simulink model "chap7_2sim_Sfunction"  (R2014b)
settings: Solver=ode45  StartTime=0.0  StopTime=10  RelTol=1e-3
libraries: fod x2
settings Model: ExtModeTrigMode=oneshot  ExtModeArmWhenConnect=off  Creator=Administrator  LastModifiedBy=Administrator
settings DataIOCC: LimitDataPoints=off  SignalLoggingSaveFormat=ModelDataLogs  SignalLoggingName=sigsOut
settings OptimizationCC: BooleanDataType=off
settings DebuggingCC: SaveWithParameterizedLinksMsg=none  UnderspecifiedInitializationDetection=Classic  MergeDetectMultiDrivingBlocksExec=none  SignalResolutionControl=TryResolveAllWithWarning  SolverPrmCheckMsg=none  MultiTaskDSMMsg=warning  MultiTaskCondExecSysMsg=none
settings HardwareCC: TargetUnknown=on
settings RTWCC: IncludeERTFirstTime=on
settings GRTTargetCC: CombineOutputUpdateFcns=off  GRTInterface=on

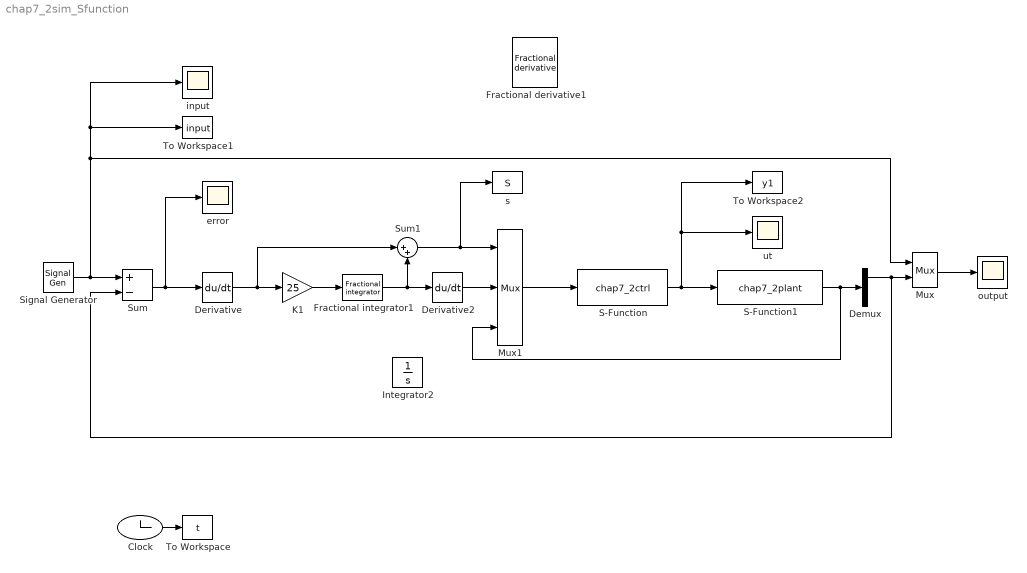
== system chap7_2sim_Sfunction ==
  Clock : Clock
  Demux : Demux  Outputs=2
  Derivative : Derivative
  Derivative2 : Derivative
  Fractional derivative1 : fod/Fractional derivative  gam=0.1  ww=[0.001; 1000]  n=5  nFod=off
  Fractional integrator1 : fod/Fractional integrator  gam=0.9  ww=[0.001; 1000]  n=3  nFod=off
  Integrator2 : Integrator
  K1 : Gain  Gain=25
  Mux : Mux  Inputs=2
  Mux1 : Mux  Inputs=3
  S-Function : S-Function  FunctionName=chap7_2ctrl  EnableBusSupport=off
  S-Function1 : S-Function  FunctionName=chap7_2plant  EnableBusSupport=off
  Signal Generator : SignalGenerator
  Sum : Sum  Inputs=+-  SaturateOnIntegerOverflow=on  InputSameDT=on  OutDataTypeStr=Inherit: Same as first input
  Sum1 : Sum  Inputs=|++
  To Workspace : ToWorkspace  VariableName=t  SampleTime=-1
  To Workspace1 : ToWorkspace  VariableName=input  SampleTime=-1
  To Workspace2 : ToWorkspace  VariableName=y1  SampleTime=-1
  error : Scope
      settings: SaveName=ScopeData2
  input : Scope
  output : Scope
  s : ToWorkspace  VariableName=S  SampleTime=-1
  ut : Scope
      settings: SaveName=ScopeData3
  wires:
  Clock/1 -> To Workspace/1
  S-Function1/1 -> Mux1/3, Demux/1
  Mux/1 -> output/1
  Sum/1 -> Derivative/1, error/1
  Signal Generator/1 -> To Workspace1/1, input/1, Mux/1, Sum/1
  S-Function/1 -> S-Function1/1, To Workspace2/1, ut/1
  Demux/1 -> Sum/2, Mux/2
  Derivative/1 -> Sum1/1, K1/1
  Sum1/1 -> s/1, Mux1/1
  K1/1 -> Fractional integrator1/1
  Fractional integrator1/1 -> Derivative2/1, Sum1/2
  Mux1/1 -> S-Function/1
  Derivative2/1 -> Mux1/2
